simulink model "modelo_SIR"  (R2019b)
settings: Solver=VariableStepAuto  StartTime=0.0  StopTime=100  RelTol=1e-3
undefined symbols (not defined in the file): beta, gamma, I0, R0, S0
settings Model: Creator=lucia  LastModifiedBy=lucia

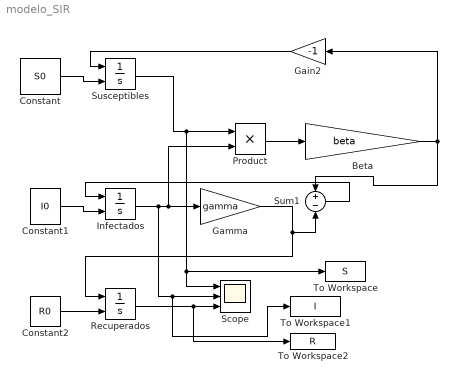
== system modelo_SIR ==
  Beta : Gain  Gain=beta
  Constant : Constant  Value=S0
  Constant1 : Constant  Value=I0
  Constant2 : Constant  Value=R0
  Gain2 : Gain  Gain=-1
  Gamma : Gain  Gain=gamma
  Infectados : Integrator  InitialConditionSource=external
  Product : Product
  Recuperados : Integrator  InitialConditionSource=external
  Scope : Scope  NumInputPorts=3
  Sum1 : Sum  Inputs=+-
  Susceptibles : Integrator  InitialConditionSource=external
  To Workspace : ToWorkspace  VariableName=S  SaveFormat=Structure With Time  SampleTime=-1
  To Workspace1 : ToWorkspace  VariableName=I  SaveFormat=Structure With Time  SampleTime=-1
  To Workspace2 : ToWorkspace  VariableName=R  SaveFormat=Structure With Time  SampleTime=-1
  wires:
  Constant/1 -> Susceptibles/2
  Constant1/1 -> Infectados/2
  Constant2/1 -> Recuperados/2
  Susceptibles/1 -> To Workspace/1, Scope/1, Product/1
  Infectados/1 -> To Workspace1/1, Scope/2, Product/2, Gamma/1
  Product/1 -> Beta/1
  Beta/1 -> Gain2/1, Sum1/1
  Sum1/1 -> Infectados/1
  Recuperados/1 -> To Workspace2/1, Scope/3
  Gamma/1 -> Recuperados/1, Sum1/2
  Gain2/1 -> Susceptibles/1
